simulink model "singlephaseinverter_DC_AC_Converter"  (R2019a)
settings: Solver=VariableStepAuto  StartTime=0.0  StopTime=10.0  RelTol=1e-3
libraries: powerlib x11, powerlib_meascontrol x3, simulink x2
settings Model: Creator=Administrator  LastModifiedBy=Administrator

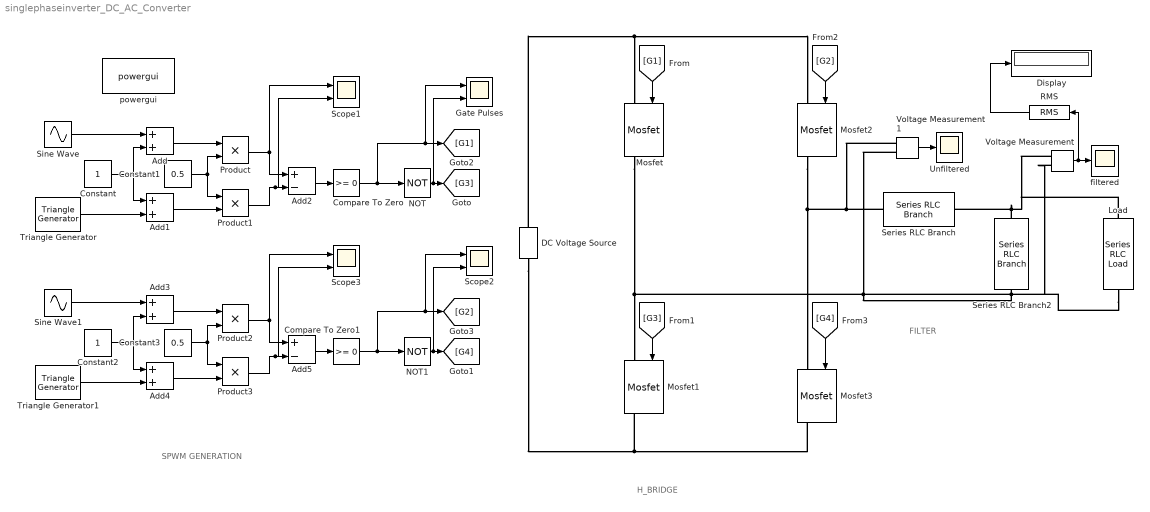
== system singlephaseinverter_DC_AC_Converter ==
  note: SPWM GENERATION
  note: H_BRIDGE
  note: FILTER
  Add{,1,3..4} (4 alike) : Sum
  Add2 : Sum  Inputs=+-
  Add5 : Sum  Inputs=+-
  Compare To Zero : simulink/Logic and Bit Operations/Compare To Zero  relop=>=  OutDataTypeStr=boolean
  Compare To Zero1 : simulink/Logic and Bit Operations/Compare To Zero  relop=>=  OutDataTypeStr=boolean
  Constant : Constant
  Constant1 : Constant  Value=0.5
  Constant2 : Constant
  Constant3 : Constant  Value=0.5
  DC Voltage Source : powerlib/Electrical Sources/DC Voltage Source  Amplitude=312  Measurements=None
      settings: SourceProductName=Simscape Electrical
  Display : Display
  Gate Pulses : Scope  NumInputPorts=2
  Load : powerlib/Elements/Series RLC Load  LConnTagsString=a  RConnTagsString=__new0  NominalVoltage=220  NominalFrequency=50  ActivePower=1e3  InductivePower=0  CapacitivePower=0  Setx0=off  InitialVoltage=0  SetiL0=off  InitialCurrent=0  Measurements=None  LoadType=constant Z
      settings: SourceProductName=Simscape Electrical
  Mosfet{,1..3} (4 alike) : powerlib/Power Electronics/Mosfet  Ron=0.1  Lon=0  Rd=0.01  Vfd=0  IC=0  Rs=1e5  Cs=inf  Measurements=on
      settings: SourceProductName=Simscape Electrical
  NOT : Logic  Operator=NOT  IconShape=distinctive  AllPortsSameDT=off  OutDataTypeStr=boolean
  NOT1 : Logic  Operator=NOT  IconShape=distinctive  AllPortsSameDT=off  OutDataTypeStr=boolean
  Product{,1..3} (4 alike) : Product
  RMS : powerlib_meascontrol/Measurements/RMS  TrueRMS=on  Freq=50  RMSInit=220  Ts=0
      settings: SourceProductName=Simscape Electrical
  Scope1 : Scope  NumInputPorts=2
  Scope2 : Scope  NumInputPorts=2
  Scope3 : Scope  NumInputPorts=2
  Series RLC Branch : powerlib/Elements/Series RLC Branch  LConnTagsString=__new0  RConnTagsString=__new0  BranchType=L  Resistance=1  Inductance=0.6e-3  SetiL0=off  InitialCurrent=0  Capacitance=1e-6  Setx0=off  InitialVoltage=0  Measurements=None
      settings: SourceProductName=Simscape Electrical
  Series RLC Branch2 : powerlib/Elements/Series RLC Branch  LConnTagsString=__new0  RConnTagsString=__new0  BranchType=C  Resistance=1  Inductance=1e-3  SetiL0=off  InitialCurrent=0  Capacitance=10000e-6  Setx0=off  InitialVoltage=0  Measurements=None
      settings: SourceProductName=Simscape Electrical
  Sine Wave : Sin  Frequency=2*pi*50  SampleTime=0
  Sine Wave1 : Sin  Frequency=2*pi*50  Phase=pi/2  SampleTime=0
  Triangle Generator : powerlib_meascontrol/Pulse & Signal Generators/Triangle Generator  Freq=1e3  Phase=0  Ts=0
      settings: SourceProductName=Simscape Electrical
  Triangle Generator1 : powerlib_meascontrol/Pulse & Signal Generators/Triangle Generator  Freq=1e3  Phase=0  Ts=0
      settings: SourceProductName=Simscape Electrical
  Unfiltered : Scope
  Voltage Measurement : powerlib/Measurements/Voltage Measurement  PhasorSimulation=off  OutputType=Complex  PSBequivalent=0
      settings: SourceProductName=Simscape Electrical
  Voltage Measurement1 : powerlib/Measurements/Voltage Measurement  PhasorSimulation=off  OutputType=Complex  PSBequivalent=0
      settings: SourceProductName=Simscape Electrical
  filtered : Scope
  powergui : powerlib/powergui  Priority=1  SimulationMode=Continuous  SampleTime=50e-6  frequency=60  Iterations=50  frequencyindice=0  Pbase=100e6  ErrMax=1e-4  UnitsV=kV  UnitsW=MW  buscounter=0  FunctionMessages=off  echomessages=off  EnableUseOfTLC=off  CurrentSourceSwitches=off  DisableSnubberDevices=off  DisableRonSwitches=off  DisableVfSwitches=off  DisplayEquations=off  AutomaticDiscreteSolvers=off  SolverType=Tustin/Backward Euler (TBE)  Interpol=off  ExternalGateDelay=off  methode=off  Ts=100  x0status=blocks  SPID=on  SwTol=0  HookPort=off  NonlinearTolerance=0  nMaxIteration=15  ContinueOnMaxIteration=off  RestoreLinks=warning  ResistiveCurrentMeasurement=off  Frange=[0:2:500]  Ylog=off  Xlog=on  ShowGrid=off  save=off  variable=ZData  structure=0  ZoomFFT=off  StartTime=0.0  cycles=1  DisplayStyle=1  fundamental=60  FreqAxis=off  MaxFrequency=1000  frequencyindicesteady=1  RmsSteady=1  display=off
      settings: SourceProductName=Simscape Electrical
  wires:
  Sine Wave/1 -> Add/1
  Constant/1 -> Add/2, Add1/1
  Triangle Generator/1 -> Add1/2
  Add2/1 -> Compare To Zero/1
  Compare To Zero/1 -> Gate Pulses/1, [G1], NOT/1
  NOT/1 -> Gate Pulses/2, [G3]
  [G1] -> Mosfet/1
  [G3] -> Mosfet1/1
  [G2] -> Mosfet2/1
  [G4] -> Mosfet3/1
  Add/1 -> Product/1
  Add1/1 -> Product1/2
  Constant1/1 -> Product1/1, Product/2
  Product/1 -> Scope1/1, Add2/1
  Product1/1 -> Scope1/2, Add2/2
  Product3/1 -> Add5/2, Scope3/2
  Product2/1 -> Add5/1, Scope3/1
  Constant3/1 -> Product2/2, Product3/1
  Add4/1 -> Product3/2
  Add3/1 -> Product2/1
  NOT1/1 -> [G4], Scope2/2
  Compare To Zero1/1 -> NOT1/1, [G2], Scope2/1
  Add5/1 -> Compare To Zero1/1
  Triangle Generator1/1 -> Add4/2
  Constant2/1 -> Add4/1, Add3/2
  Sine Wave1/1 -> Add3/1
  Voltage Measurement/1 -> RMS/1, filtered/1
  Voltage Measurement1/1 -> Unfiltered/1
  RMS/1 -> Display/1
  connections:
  DC Voltage Source/RConn1 -- Mosfet/LConn1 -- Mosfet2/LConn1
  DC Voltage Source/LConn1 -- Mosfet1/RConn1 -- Mosfet3/RConn1
  Series RLC Branch2/LConn1 -- Voltage Measurement/LConn1 -- Load/LConn1 -- Series RLC Branch/RConn1
  Mosfet/RConn1 -- Voltage Measurement1/LConn2 -- Series RLC Branch2/RConn1 -- Load/RConn1 -- Voltage Measurement/LConn2 -- Mosfet1/LConn1
  Voltage Measurement1/LConn1 -- Series RLC Branch/LConn1 -- Mosfet3/LConn1 -- Mosfet2/RConn1
